simulink model "plant1_start_2_3"  (R2018a)
settings: Solver=FixedStepAuto  StartTime=0.0  StopTime=10.0  FixedStep=0.01  RelTol=1e-3
settings Model: Creator=anike  LastModifiedBy=anike
settings DebuggingCC: RootOutportRequireBusObject=error  StrictBusMsg=ErrorOnBusTreatedAsVector
settings HardwareCC: ProdBitPerPointer=32  ProdBitPerSizeT=32  ProdBitPerPtrDiffT=32  ProdLargestAtomicFloat=None  ProdWordSize=32  ProdHWDeviceType=Intel->x86/Pentium
settings RTWCC: SystemTargetFile=NIVeriStand.tlc  TemplateMakefile=NIVeriStand_vc.tmf  Description=NI Phar Lap Real-Time & Windows Targets  TargetLang=C++
settings STFCustomTargetCC: TargetLangStandard=C++03 (ISO)  MatFileLogging=on  SystemTargetFile=NIVeriStand.tlc
settings GRTTargetCC: TargetLangStandard=C++03 (ISO)  ParMdlRefBuildCompliant=off  CompOptLevelCompliant=off  ConcurrentExecutionCompliant=off  CombineOutputUpdateFcns=off  CPPClassGenCompliant=off  GRTInterface=on  UseToolchainInfoCompliant=off

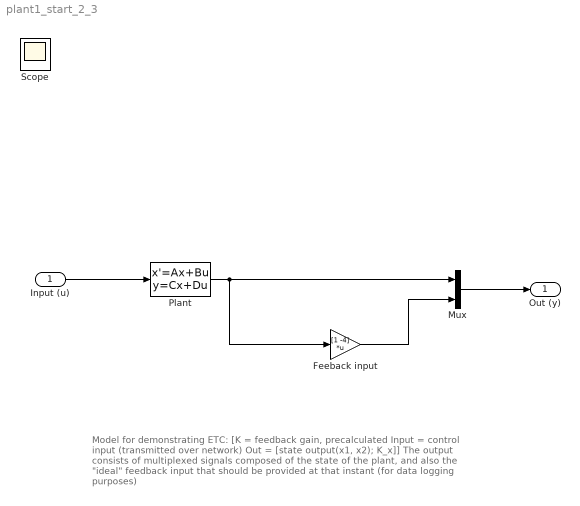
== system plant1_start_2_3 ==
  note: Model for demonstrating ETC:
      |
      | [K = feedback gain, precalculated
      | Input = control input (transmitted over network)
      | Out = [state output(x1, x2); K_x]]
      |
      | The output consists of multiplexed signals composed of the state of the plant, and also the "ideal" feedback input that should be provided at that instant (for data logging purposes)
  "Input (u) " : Inport
  Feeback input : Gain  Gain=[1 -4]  Multiplication=Matrix(K*u)
  Mux : Mux  Inputs=2
  Plant : StateSpace  A=[0 1; -2 3]  B=[0; 1]  C=[1 0; 0 1]  D=[0; 0]  InitialCondition=[2 3]
  Out (y) : Outport
  Scope : Scope
  wires:
  Plant/1 -> Mux/1, Feeback input/1
  "Input (u) "/1 -> Plant/1
  Mux/1 -> Out (y)/1
  Feeback input/1 -> Mux/2
